simulink model "BESS_Voltage_Controle"  (R2017b)
settings: Solver=ode45  StartTime=0.0  StopTime=5  RelTol=1e-3  EnableMultiTasking=on
values from neighbouring files (symbols this model uses):
  beta = beta (k)    [Parameter_2M_DFIG_BESS.m]
  Cbus = 80e-3    (= 0.08)    [Parameter_2M_DFIG_BESS.m]
  cp_opt_abs = abs(max(Cp))    [Parameter_2M_DFIG_BESS.m]
  D = 0.1    [Parameter_2M_DFIG_BESS.m]
  f = 60    [Parameter_2M_DFIG_BESS.m]
  Fs = 1.8    [Parameter_2M_DFIG_BESS.m]
  fsw = 4e3    (= 4000)    [Parameter_2M_DFIG_BESS.m]
  J = 90    [Parameter_2M_DFIG_BESS.m]
  ki_id = (wni^2)*Lr*sigma    (= 491.599501999)    [Parameter_2M_DFIG_BESS.m]
  ki_idg = (wnig^2)*Lg    (= 68.6450725305)    [Parameter_2M_DFIG_BESS.m]
  ki_iq = ki_id    (= 491.599501999)    [Parameter_2M_DFIG_BESS.m]
  ki_iqg = ki_idg    (= 68.6450725305)    [Parameter_2M_DFIG_BESS.m]
  ki_v = -300000    [Parameter_2M_DFIG_BESS.m]
  kp_id = (2*wni*sigma*Lr)-Rr    (= 0.5771)    [Parameter_2M_DFIG_BESS.m]
  kp_idg = (2*wnig*Lg)-Rg    (= 0.364153420404)    [Parameter_2M_DFIG_BESS.m]
  kp_iq = kp_id    (= 0.5771)    [Parameter_2M_DFIG_BESS.m]
  kp_iqg = kp_idg    (= 0.364153420404)    [Parameter_2M_DFIG_BESS.m]
  kp_v = -1000    [Parameter_2M_DFIG_BESS.m]
  Kpg = 1/(1.5*Vs*sqrt(2/3))    [Parameter_2M_DFIG_BESS.m]
  Kqg = -Kpg    [Parameter_2M_DFIG_BESS.m]
  lambda_opt = abs(lambda(posicion))    [Parameter_2M_DFIG_BESS.m]
  Lg = 483e-6    (= 0.000483)    [Parameter_2M_DFIG_BESS.m]
  Lm = 2.5e-3    (= 0.0025)    [Parameter_2M_DFIG_BESS.m]
  Lr = Lm + Lsr    (= 0.002587)    [Parameter_2M_DFIG_BESS.m]
  Ls = Lm + Lsi    (= 0.002587)    [Parameter_2M_DFIG_BESS.m]
  Lsi = 87e-6    (= 8.7e-05)    [Parameter_2M_DFIG_BESS.m]
  N = 100    [Parameter_2M_DFIG_BESS.m]
  p = 2    [Parameter_2M_DFIG_BESS.m]
  Ps = 2e6    (= 2000000)    [Parameter_2M_DFIG_BESS.m]
  Radio = 44    [Parameter_2M_DFIG_BESS.m]
  Rg = 20e-6    (= 2e-05)    [Parameter_2M_DFIG_BESS.m]
  ro = 1.225    [Parameter_2M_DFIG_BESS.m]
  Rr = 2.9e-3    (= 0.0029)    [Parameter_2M_DFIG_BESS.m]
  Rs = 2.6e-3    (= 0.0026)    [Parameter_2M_DFIG_BESS.m]
  sigma = 1- Lm^2/(Ls*Lr)    (= 0.0661284179513)    [Parameter_2M_DFIG_BESS.m]
  Ts = 1/fsw/f    (= 4.16666666667e-06)    [Parameter_2M_DFIG_BESS.m]
  Vbus_ref = 1200    [Parameter_2M_DFIG_BESS.m]
  Vs = 690    [Parameter_2M_DFIG_BESS.m]
undefined symbols (not defined in the file or in its folder): D1, D11, Delta, DiscIntNeverNeededParam, Ion, Lithium, sigbuilder_block
libraries: powerlib x50, powerlib_meascontrol x21, electricdrivelib x1, simulink x1, sps_avr x1
(part 1 of 2)
settings Model: SimulationMode=accelerator  Creator=admin  LastModifiedBy=admin
settings DataIOCC: LimitDataPoints=on  SaveFormat=Array
settings OptimizationCC: EfficientMapNaN2IntZero=off  LifeSpan=inf
settings DebuggingCC: UnderspecifiedInitializationDetection=Classic  MergeDetectMultiDrivingBlocksExec=none  SolverPrmCheckMsg=warning  StateNameClashWarn=warning  SFUnexpectedBacktrackingDiag=warning  SFNoUnconditionalDefaultTransitionDiag=warning  SFExecutionAtInitializationDiag=none
settings HardwareCC: ProdBitPerPointer=32  ProdBitPerSizeT=32  ProdBitPerPtrDiffT=32  ProdLargestAtomicFloat=None  ProdIntDivRoundTo=Undefined  ProdEndianess=Unspecified  ProdWordSize=32  ProdHWDeviceType=32-bit Generic  TargetBitPerPointer=64  TargetBitPerSizeT=64  TargetBitPerPtrDiffT=64  TargetLongLongMode=on  TargetIntDivRoundTo=Zero  TargetEndianess=LittleEndian  TargetWordSize=64  TargetHWDeviceType=MATLAB Host  ProdEqTarget=off
settings ModelReferenceCC: PropagateSignalLabelsOutOfModel=off
settings CodeAppCC: MaxIdLength=128
settings GRTTargetCC: TargetLangStandard=C89/C90 (ANSI)  CombineOutputUpdateFcns=off  GRTInterface=on
settings ConfigComp: CovMetricSettings=dw  CovHtmlReporting=on  CovSaveCumulativeToWorkspaceVar=on  CovSaveSingleToWorkspaceVar=on  CovExternalEMLEnable=off
settings SimscapeCC: SimscapeNormalizeSystem=off

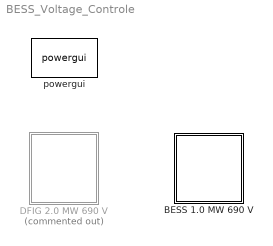
== system BESS_Voltage_Controle ==
  BESS 1.0 MW 690 V : Subsystem
  DFIG 2.0 MW 690 V : Subsystem  Commented=on
  powergui : powerlib/powergui  Priority=1  SimulationMode=Discrete  SampleTime=Ts  frequency=60  Iterations=50  frequencyindice=0  Pbase=100e6  ErrMax=1e-4  UnitsV=kV  UnitsW=MW  buscounter=0  FunctionMessages=off  echomessages=off  EnableUseOfTLC=off  CurrentSourceSwitches=off  DisableSnubberDevices=off  DisableRonSwitches=off  DisableVfSwitches=off  DisplayEquations=off  SolverType=Tustin  Interpol=off  ExternalGateDelay=off  methode=off  Ts=0  x0status=blocks  SPID=off  SwTol=0  HookPort=off  RestoreLinks=warning  ResistiveCurrentMeasurement=off  Frange=[0:2:500]  Ylog=off  Xlog=on  ShowGrid=off  save=off  variable=ZData  structure=0  ZoomFFT=off  StartTime=0.0  cycles=1  DisplayStyle=1  fundamental=60  FreqAxis=off  MaxFrequency=1000  frequencyindicesteady=1  RmsSteady=1  display=off

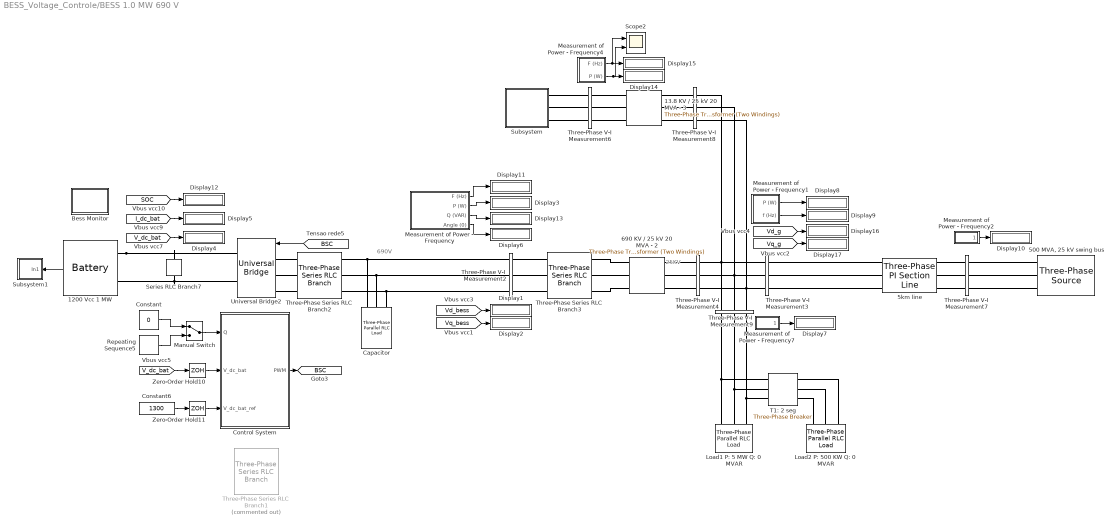
== system BESS_Voltage_Controle/BESS 1.0 MW 690 V ==
  note: 690V
  note: 25KV
  "1200 Vcc 1 MW " : electricdrivelib/Extra Sources/Battery  BatType=Lithium-Ion  ShowTempParam=off  ThermalPreset=no  ShowAgeParam=off  NomV=1200  NomQ=833  SOC=71  Batt_Tr=30  PresetModel=on  MaxQ=833  MinV=900  FullV=1396.7846  Dis_rate=362.1739  R=0.014406  Normal_OP=753.3217  expZone="[1296.463      40.925652]"  current=[833]  Units=Time  Tci=20  NomT=25  T2=0  MaxQ2=2.208  FullV2=3.45  Normal_OP2=2.8  expZone2="[3.22        0.23]"  Rca=0.6  ti=1000  Dp=0  Neq0=0  Tsim=1e6  Ta1=25  Qeol=5.4*0.9  Reol=0.013333*1.2  Char_age=[2.3478, 3]  Dis_age=[2.3478, 10]  N1=1500  N2=10500  N3=1000  N4=1400  Ta2=45  N5=950
  13.8 KV / 25 kV 20 MVA - 3 : powerlib/Elements/Three-Phase Transformer (Two Windings)  Winding1Connection=Delta (D11)  Winding2Connection=Yg  CoreType=Three single-phase transformers  SetSaturation=off  Hysteresis=off  DataFile='hysteresis'  SetInitialFlux=off  Measurements=None  UNITS=SI  NominalPower=[20e6 f]  Winding1=[25000 0.14881 0.011842]  Winding2=[13800 2.624e-05 2.0881e-06]  Rm=89286  Lm=Inf  L0=0.5  Saturation=[0 0;0.47518 112.54;197.99 142.55]  InitialFluxes=[75.026 -75.026 65.648]  MoreParameters=off  BreakLoop=off  DataType=on  TransfoNumber=0
  "500 MVA, 25 kV swing bus" : powerlib/Electrical Sources/Three-Phase Source  InternalConnection=Yg  VoltagePhases=off  Voltage=25e3  PhaseAngle=0  Voltage_phases=[25e3 25e3 25e3]/sqrt(3)  PhaseAngles_phases=[0 -120 +120]  Frequency=f  NonIdealSource=on  SpecifyImpedance=on  Resistance=0  Inductance=47.147e-3  ShortCircuitLevel=500e6  BaseVoltage=25e3  XRratio=100  BusType=swing  Pref=10e3  Qref=0  Prefabc=[10e3, 10e3, 10e3]  Qrefabc=[0, 0, 0]  Qmin=-inf  Qmax=inf
  5km line : powerlib/Elements/Three-Phase PI Section Line  LConnTagsString=a|b|c  RConnTagsString=A|B|C  Frequency=f  Resistances=[0.1153 0.413]  Inductances=[1.05e-3 3.32e-3]  Capacitances=[11.33e-009 5.01e-009]  Length=5
      settings: SourceProductName=Simscape Power Systems
  690 KV / 25 kV 20 MVA - 2 : powerlib/Elements/Three-Phase Transformer (Two Windings)  Winding1Connection=Delta (D11)  Winding2Connection=Yg  CoreType=Three single-phase transformers  SetSaturation=off  Hysteresis=off  DataFile='hysteresis'  SetInitialFlux=off  Measurements=None  UNITS=SI  NominalPower="[20e6  f]"  Winding1=[25000 0.14881 0.011842]  Winding2=[690 2.624e-05 2.0881e-06]  Rm=89286  Lm=Inf  L0=0.5  Saturation=[0 0;0.47518 112.54;197.99 142.55]  InitialFluxes=[75.026 -75.026 65.648]  MoreParameters=off  BreakLoop=off  DataType=on  TransfoNumber=0
  Bess Monitor : Subsystem
  Capacitor : powerlib/Elements/Three-Phase Parallel RLC Load  LConnTagsString=A|B|C  Configuration=Y (grounded)  NominalVoltage=690  Vabc=[1e3 1e3 1e3]  Vabcp=[1e3 1e3 1e3]  NominalFrequency=f  UnbalancedPower=off  ActivePower=0  InductivePower=0  CapacitivePower=15e-3  Pabc=[10e3 9e3 11e3]  QLabc=[100 90 110]  QCabc=[100 90 110]  Pabcp=[10e3 9e3 11e3]  QLabcp=[100 90 110]  QCabcp=[100 90 110]  Measurements=None  LoadType=constant Z
  Constant : Constant  Value=0
  Constant6 : Constant  Value=1300
  Control System : Subsystem
  Display{1..17} (17 alike) : Display
  Load1 P: 5 MW Q: 0 MVAR : powerlib/Elements/Three-Phase Parallel RLC Load  LConnTagsString=A|B|C  Configuration=Y (grounded)  NominalVoltage=25e3  Vabc=[1e3 1e3 1e3]  Vabcp=[1e3 1e3 1e3]  NominalFrequency=f  UnbalancedPower=off  ActivePower=5e6  InductivePower=0  CapacitivePower=0  Pabc=[10e3 9e3 11e3]  QLabc=[100 90 110]  QCabc=[100 90 110]  Pabcp=[10e3 9e3 11e3]  QLabcp=[100 90 110]  QCabcp=[100 90 110]  Measurements=None  LoadType=constant I
  Load2 P: 500 KW Q: 0 MVAR : powerlib/Elements/Three-Phase Parallel RLC Load  LConnTagsString=A|B|C  Configuration=Y (grounded)  NominalVoltage=25e3  Vabc=[1e3 1e3 1e3]  Vabcp=[1e3 1e3 1e3]  NominalFrequency=f  UnbalancedPower=off  ActivePower=500e5  InductivePower=0  CapacitivePower=0  Pabc=[10e3 9e3 11e3]  QLabc=[100 90 110]  QCabc=[100 90 110]  Pabcp=[10e3 9e3 11e3]  QLabcp=[100 90 110]  QCabcp=[100 90 110]  Measurements=None  LoadType=constant I
  Manual Switch : ManualSwitch
  Measurement of Power - Frequency : Subsystem
  Measurement of Power - Frequency1 : Subsystem
  Measurement of Power - Frequency2 : Subsystem
  Measurement of Power - Frequency4 : Subsystem
  Measurement of Power - Frequency7 : Subsystem
  Repeating Sequence5 : simulink/Sources/Repeating Sequence  rep_seq_t=[0 1.499 1.5 2.499 2.5 3.499 3.5 3.999 4 5]  rep_seq_y=[0 0 5e5 5e5 3e5 3e5 -5e5 -5e5 0 0]
  Scope2 : Scope  NumInputPorts=2
  Series RLC Branch7 : powerlib/Elements/Series RLC Branch  LConnTagsString=__new0  RConnTagsString=__new0  BranchType=C  Resistance=1  Inductance=1e-3  SetiL0=off  InitialCurrent=0  Capacitance=15e-3  Setx0=off  InitialVoltage=0  Measurements=Branch voltage
  Subsystem : Subsystem
  Subsystem1 : Subsystem
  "T1: 2 seg " : powerlib/Elements/Three-Phase Breaker  InitialState=open  SwitchA=on  SwitchB=on  SwitchC=on  SwitchTimes=5  External=off  BreakerResistance=0.01  SnubberResistance=1e6  SnubberCapacitance=inf  Measurements=None
  Three-Phase Series RLC Branch1 : powerlib/Elements/Three-Phase Series RLC Branch  Commented=on  LConnTagsString=A|B|C  RConnTagsString=A|B|C  BranchType=RL  Resistance=20e-6  Inductance=483e-6  Capacitance=0  Measurements=None
  Three-Phase Series RLC Branch2 : powerlib/Elements/Three-Phase Series RLC Branch  LConnTagsString=A|B|C  RConnTagsString=A|B|C  BranchType=RL  Resistance=20e-3  Inductance=483e-6  Capacitance=0  Measurements=None
  Three-Phase Series RLC Branch3 : powerlib/Elements/Three-Phase Series RLC Branch  LConnTagsString=A|B|C  RConnTagsString=A|B|C  BranchType=RL  Resistance=20e-3  Inductance=0  Capacitance=0  Measurements=None
  Three-Phase V-I Measurement2 : powerlib/Measurements/Three-Phase V-I Measurement  VoltageMeasurement=phase-to-ground  SetLabelV=on  LabelV=V_ac_bess  Vpu=off  VpuLL=off  CurrentMeasurement=yes  SetLabelI=on  LabelI=I_ac_bess  Ipu=off  Pbase=100e6  Vbase=500e3  OutputType=Complex  PhasorSimulation=off  PSBequivalent=0
  Three-Phase V-I Measurement3 : powerlib/Measurements/Three-Phase V-I Measurement  VoltageMeasurement=phase-to-ground  SetLabelV=on  LabelV=V_ac_line_1  Vpu=off  VpuLL=off  CurrentMeasurement=yes  SetLabelI=on  LabelI=I_ac_line_1  Ipu=off  Pbase=100e6  Vbase=500e3  OutputType=Complex  PhasorSimulation=off  PSBequivalent=0
  Three-Phase V-I Measurement4 : powerlib/Measurements/Three-Phase V-I Measurement  VoltageMeasurement=phase-to-ground  SetLabelV=on  LabelV=V_ac_bat_H  Vpu=off  VpuLL=off  CurrentMeasurement=yes  SetLabelI=on  LabelI=I_ac_bat_H  Ipu=off  Pbase=100e6  Vbase=500e3  OutputType=Complex  PhasorSimulation=off  PSBequivalent=0
  Three-Phase V-I Measurement6 : powerlib/Measurements/Three-Phase V-I Measurement  VoltageMeasurement=phase-to-ground  SetLabelV=on  LabelV=V_ac_syn_low  Vpu=off  VpuLL=off  CurrentMeasurement=yes  SetLabelI=on  LabelI=I_ac_syn_low  Ipu=off  Pbase=100e6  Vbase=500e3  OutputType=Complex  PhasorSimulation=off  PSBequivalent=0
  Three-Phase V-I Measurement7 : powerlib/Measurements/Three-Phase V-I Measurement  VoltageMeasurement=phase-to-ground  SetLabelV=on  LabelV=V_ac_line_2  Vpu=off  VpuLL=off  CurrentMeasurement=yes  SetLabelI=on  LabelI=I_ac_line_2  Ipu=off  Pbase=100e6  Vbase=500e3  OutputType=Complex  PhasorSimulation=off  PSBequivalent=0
  Three-Phase V-I Measurement8 : powerlib/Measurements/Three-Phase V-I Measurement  VoltageMeasurement=phase-to-ground  SetLabelV=on  LabelV=V_ac_syn_H  Vpu=off  VpuLL=off  CurrentMeasurement=yes  SetLabelI=on  LabelI=I_ac_syn_H  Ipu=off  Pbase=100e6  Vbase=500e3  OutputType=Complex  PhasorSimulation=off  PSBequivalent=0
  Three-Phase V-I Measurement9 : powerlib/Measurements/Three-Phase V-I Measurement  VoltageMeasurement=phase-to-ground  SetLabelV=on  LabelV=V_ac_load  Vpu=off  VpuLL=off  CurrentMeasurement=yes  SetLabelI=on  LabelI=I_ac_load  Ipu=off  Pbase=100e6  Vbase=500e3  OutputType=Complex  PhasorSimulation=off  PSBequivalent=0
  Universal Bridge2 : powerlib/Power Electronics/Universal Bridge  Arms=3  SnubberResistance=1e5  SnubberCapacitance=inf  Device=Ideal Switches  Ron=1e-3  Lon=0  ForwardVoltages="[  0  0  ]"  ForwardVoltage=0  GTOparameters=[ 10e-6 , 20e-6 ]  IGBTparameters=[ 1e-6 , 2e-6 ]  Measurements=None  Measurements_2=None  converterType=Rectifier
  Zero-Order Hold10 : ZeroOrderHold  SampleTime=1/fsw
  Zero-Order Hold11 : ZeroOrderHold  SampleTime=1/fsw
  tag scope: BSC=global
  wires:
  Zero-Order Hold10/1 -> Control System/2(V_dc_bat)
  [V_dc_bat] -> Zero-Order Hold10/1
  [I_dc_bat] -> Display5/1
  Control System/1(PWM) -> [BSC]
  Zero-Order Hold11/1 -> Control System/3(V_dc_bat_ref)
  [V_dc_bat] -> Display4/1
  "1200 Vcc 1 MW "/1 -> Subsystem1/1(In1)
  Constant6/1 -> Zero-Order Hold11/1
  [BSC] -> Universal Bridge2/1
  Measurement of Power - Frequency/2(P (W)) -> Display3/1
  Measurement of Power - Frequency/1(F (Hz)) -> Display11/1
  Measurement of Power - Frequency/3(Q (VAR)) -> Display13/1
  [SOC] -> Display12/1
  Manual Switch/1 -> Control System/1(Q)
  Constant/1 -> Manual Switch/1
  Repeating Sequence5/1 -> Manual Switch/2
  [Vd_bess] -> Display1/1
  [Vq_bess] -> Display2/1
  Measurement of Power - Frequency/4(Angle (0)) -> Display6/1
  Measurement of Power - Frequency7/1(P (W)) -> Display7/1
  Measurement of Power - Frequency2/1(P (W)) -> Display10/1
  Measurement of Power - Frequency1/1(P (W)) -> Display8/1
  Measurement of Power - Frequency4/2(P (W)) -> Display14/1, Scope2/2
  Measurement of Power - Frequency4/1(F (Hz)) -> Scope2/1, Display15/1
  [Vd_g] -> Display16/1
  [Vq_g] -> Display17/1
  Measurement of Power - Frequency1/2(f (Hz)) -> Display9/1
  connections:
  Series RLC Branch7/RConn1 -- "1200 Vcc 1 MW "/LConn2 -- Universal Bridge2/RConn2
  "1200 Vcc 1 MW "/LConn1 -- Series RLC Branch7/LConn1 -- Universal Bridge2/RConn1
  Capacitor/LConn1 -- Three-Phase V-I Measurement2/LConn1 -- Three-Phase Series RLC Branch2/RConn1
  Capacitor/LConn2 -- Three-Phase Series RLC Branch2/RConn2 -- Three-Phase V-I Measurement2/LConn2
  Capacitor/LConn3 -- Three-Phase V-I Measurement2/LConn3 -- Three-Phase Series RLC Branch2/RConn3
  Load1 P: 5 MW Q: 0 MVAR/LConn1 -- Three-Phase V-I Measurement9/RConn3 -- "T1: 2 seg "/LConn1
  Load1 P: 5 MW Q: 0 MVAR/LConn2 -- Three-Phase V-I Measurement9/RConn2 -- "T1: 2 seg "/LConn2
  Load1 P: 5 MW Q: 0 MVAR/LConn3 -- Three-Phase V-I Measurement9/RConn1 -- "T1: 2 seg "/LConn3
  690 KV / 25 kV 20 MVA - 2/LConn2 -- Three-Phase V-I Measurement4/LConn2
  690 KV / 25 kV 20 MVA - 2/LConn3 -- Three-Phase V-I Measurement4/LConn3
  690 KV / 25 kV 20 MVA - 2/LConn1 -- Three-Phase V-I Measurement4/LConn1
  5km line/RConn1 -- Three-Phase V-I Measurement7/LConn1
  5km line/LConn1 -- Three-Phase V-I Measurement3/RConn1
  5km line/LConn2 -- Three-Phase V-I Measurement3/RConn2
  5km line/RConn2 -- Three-Phase V-I Measurement7/LConn2
  5km line/RConn3 -- Three-Phase V-I Measurement7/LConn3
  5km line/LConn3 -- Three-Phase V-I Measurement3/RConn3
  "500 MVA, 25 kV swing bus"/RConn1 -- Three-Phase V-I Measurement7/RConn1
  "500 MVA, 25 kV swing bus"/RConn2 -- Three-Phase V-I Measurement7/RConn2
  "500 MVA, 25 kV swing bus"/RConn3 -- Three-Phase V-I Measurement7/RConn3
  Three-Phase V-I Measurement4/RConn1 -- Three-Phase V-I Measurement8/RConn1 -- Three-Phase V-I Measurement9/LConn3 -- Three-Phase V-I Measurement3/LConn1
  Three-Phase V-I Measurement4/RConn2 -- Three-Phase V-I Measurement8/RConn2 -- Three-Phase V-I Measurement9/LConn2 -- Three-Phase V-I Measurement3/LConn2
  Three-Phase V-I Measurement4/RConn3 -- Three-Phase V-I Measurement8/RConn3 -- Three-Phase V-I Measurement3/LConn3 -- Three-Phase V-I Measurement9/LConn1
  Load2 P: 500 KW Q: 0 MVAR/LConn1 -- "T1: 2 seg "/RConn3
  Load2 P: 500 KW Q: 0 MVAR/LConn2 -- "T1: 2 seg "/RConn2
  Load2 P: 500 KW Q: 0 MVAR/LConn3 -- "T1: 2 seg "/RConn1
  Subsystem/LConn2 -- Three-Phase V-I Measurement6/LConn2
  Three-Phase V-I Measurement8/LConn3 -- 13.8 KV / 25 kV 20 MVA - 3/LConn3
  Subsystem/LConn3 -- Three-Phase V-I Measurement6/LConn3
  Subsystem/LConn1 -- Three-Phase V-I Measurement6/LConn1
  Three-Phase V-I Measurement8/LConn2 -- 13.8 KV / 25 kV 20 MVA - 3/LConn2
  Three-Phase V-I Measurement6/RConn3 -- 13.8 KV / 25 kV 20 MVA - 3/RConn3
  Three-Phase V-I Measurement6/RConn2 -- 13.8 KV / 25 kV 20 MVA - 3/RConn2
  Three-Phase V-I Measurement6/RConn1 -- 13.8 KV / 25 kV 20 MVA - 3/RConn1
  Three-Phase V-I Measurement8/LConn1 -- 13.8 KV / 25 kV 20 MVA - 3/LConn1
  Three-Phase Series RLC Branch2/LConn1 -- Universal Bridge2/LConn1
  Three-Phase Series RLC Branch2/LConn2 -- Universal Bridge2/LConn2
  Three-Phase Series RLC Branch2/LConn3 -- Universal Bridge2/LConn3
  Three-Phase Series RLC Branch3/LConn1 -- Three-Phase V-I Measurement2/RConn1
  Three-Phase Series RLC Branch3/LConn2 -- Three-Phase V-I Measurement2/RConn2
  Three-Phase Series RLC Branch3/LConn3 -- Three-Phase V-I Measurement2/RConn3
  Three-Phase Series RLC Branch3/RConn1 -- 690 KV / 25 kV 20 MVA - 2/RConn1
  Three-Phase Series RLC Branch3/RConn2 -- 690 KV / 25 kV 20 MVA - 2/RConn2
  Three-Phase Series RLC Branch3/RConn3 -- 690 KV / 25 kV 20 MVA - 2/RConn3

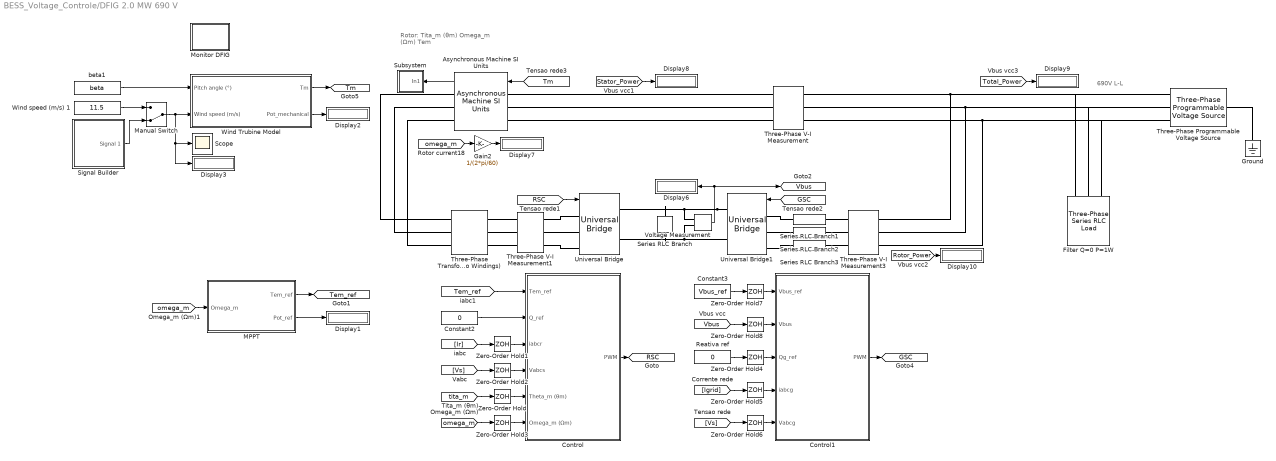
== system BESS_Voltage_Controle/DFIG 2.0 MW 690 V ==
  note: 690V L-L
  note: Rotor:
      | Tita_m (θm)
      | Omega_m (Ωm)
      | Tem
  Asynchronous Machine SI Units : powerlib/Machines/Asynchronous Machine SI Units  RotorType=Wound  PresetModel=No  MechanicalLoad=Torque Tm  ShowDetailedParameters=on  ReferenceFrame=Rotor  Units=SI  MeasurementBus=off  NominalParameters=[ Ps Vs f ]  Stator=[ Rs , Lsi]  Rotor=[ Rr , Lsi]  Cage1=[ 0.022 0.226/377]  Cage2=[ 0.022 0.226/377]  Lm=Lm  Mechanical=[ J D 2 ]  PolePairs=2  InitialConditions=[1 0 0 0 0 0 0 0]  SimulateSaturation=off  Saturation=[14.03593122, 27.81365428, 53.79336849, 72.68890987, 97.98006896, 148.6815601, 215.7428561, 302.9841135, 420.4778367 ; 230, 322, 414, 460, 506, 552, 598, 644, 690]  LoadFlowParameters=1492000  TsPowergui=0  TsBlock=-1  IterativeModel=Trapezoidal non iterative  IterativeDiscreteModel=Trapezoidal non iterative  Pmec=0
  Constant2 : Constant  Value=0
  Constant3 : Constant  Value=Vbus_ref
  Control : Subsystem
  Control1 : Subsystem
  Display{1..3,6..10} (8 alike) : Display
  Filter Q=0 P=1W : powerlib/Elements/Three-Phase Series RLC Load  LConnTagsString=A|B|C  Configuration=Y (grounded)  NominalVoltage=Vs  Vabc=[1e3 1e3 1e3]  Vabcp=[1e3 1e3 1e3]  NominalFrequency=f  UnbalancedPower=off  ActivePower=1  InductivePower=0  CapacitivePower=0  Pabc=[10e3 9e3 11e3]  QLabc=[100 90 110]  QCabc=[100 90 110]  Pabcp=[10e3 9e3 11e3]  QLabcp=[100 90 110]  QCabcp=[100 90 110]  Measurements=None  LoadType=constant Z
  Gain2 : Gain  Gain=1/(2*pi/60)
  Ground : powerlib/Elements/Ground  LConnTagsString=a
  MPPT : Subsystem
  Manual Switch : ManualSwitch  CurrentSetting=0
  Monitor DFIG : Subsystem
  Reativa ref : Constant  Value=0
  Scope : Scope
  Series RLC Branch : powerlib/Elements/Series RLC Branch  LConnTagsString=__new0  RConnTagsString=__new0  BranchType=C  Resistance=1  Inductance=1e-3  SetiL0=off  InitialCurrent=0  Capacitance=Cbus  Setx0=off  InitialVoltage=0  Measurements=Branch voltage
  Series RLC Branch1 : powerlib/Elements/Series RLC Branch  LConnTagsString=__new0  RConnTagsString=__new0  BranchType=RL  Resistance=Rg  Inductance=Lg  SetiL0=off  InitialCurrent=0  Capacitance=0  Setx0=off  InitialVoltage=0  Measurements=None
  Series RLC Branch2 : powerlib/Elements/Series RLC Branch  LConnTagsString=__new0  RConnTagsString=__new0  BranchType=RL  Resistance=Rg  Inductance=Lg  SetiL0=off  InitialCurrent=0  Capacitance=0  Setx0=off  InitialVoltage=0  Measurements=None
  Series RLC Branch3 : powerlib/Elements/Series RLC Branch  LConnTagsString=__new0  RConnTagsString=__new0  BranchType=RL  Resistance=Rg  Inductance=Lg  SetiL0=off  InitialCurrent=0  Capacitance=0  Setx0=off  InitialVoltage=0  Measurements=None
  Signal Builder : Subsystem  Tag=STV Subsys  LoadFcn=sigbuilder_block('load');  StartFcn=sigbuilder_block('start');  StopFcn=sigbuilder_block('stop');  ClipboardFcn=sigbuilder_block('clipboard');  mask(Sigbuilder block){tuvar=[0:10]}
      mask help: Simulink:masks:SigbuilderBlock_MD
      mask init:
      | if ~strcmp(get_param(bdroot(gcbh),'SimulationStatus'),'stopped') tuvar = sigbuilder_block('maskInit'); end
      settings: CopyFcn=sigbuilder_block('copy');  DeleteFcn=sigbuilder_block('delete');  ModelCloseFcn=sigbuilder_block('modelClose');  PreSaveFcn=sigbuilder_block('preSave');  PauseFcn=sigbuilder_block('pause');  ContinueFcn=sigbuilder_block('continue');  NameChangeFcn=sigbuilder_block('namechange');  OpenFcn=sigbuilder_block('open',[6 22.5 1012.5 455.25 ]);  CloseFcn=sigbuilder_block('close');
      mask Display: plot(0, 0, 100, 100,[2, 2, 32, 32, 2], [68, 8, 8, 68, 68],[32, 2], [38, 38], [32, 19, 2],[53, 60, 44], [32, 17, 17, 2],[16, 16, 31, 31]);txt = getActiveGroup(gcbh);text(2, 100, txt,'verticalAlignment', 'top');
  Subsystem : Subsystem
  Three-Phase Programmable Voltage Source : powerlib/Electrical Sources/Three-Phase Programmable Voltage Source  PositiveSequence="[Vs  0 f]"  VariationEntity=Frequency  VariationType=Table of time-amplitude pairs  VariationTypeAlt=Step  VariationStep=-0.8  VariationRate=10  VariationMagnitude=0.3  VariationFrequency=2  VariationTiming=[0.2 3]  VariationPhaseA=off  Amplitudes=[1 0.8 1.2 1.0]  TimeValues=[0 0.1 0.15 0.2]  HarmonicGeneration=off  HarmonicA=[3 0.2 -25 0]  HarmonicB=[2 0.15 35 2]  Timing="[0.05  3]"  BusType=swing  Pref=0  Qref=0  Qmin=-inf  Qmax=inf
  Three-Phase Transformer (Two Windings) : powerlib/Elements/Three-Phase Transformer (Two Windings)  Winding1Connection=Y  Winding2Connection=Y  CoreType=Three single-phase transformers  SetSaturation=off  Hysteresis=off  DataFile='hysteresis'  SetInitialFlux=off  Measurements=None  UNITS=SI  NominalPower=[ Ps , f]  Winding1=[Vs 0 0]  Winding2=[Vs/u 0 0]  Rm=1.0805e+06  Lm=2866  L0=0.5  Saturation=[0 0;0.66653 1910.3;277.72 2419.7]  InitialFluxes=[1273.5 -1273.5 1114.3]  MoreParameters=off  BreakLoop=off  DataType=on  TransfoNumber=1
  Three-Phase V-I Measurement : powerlib/Measurements/Three-Phase V-I Measurement  VoltageMeasurement=phase-to-ground  SetLabelV=on  LabelV=Vs  Vpu=off  VpuLL=off  CurrentMeasurement=yes  SetLabelI=on  LabelI=Is  Ipu=off  Pbase=100e6  Vbase=500e3  OutputType=Complex  PhasorSimulation=off  PSBequivalent=0
  Three-Phase V-I Measurement1 : powerlib/Measurements/Three-Phase V-I Measurement  VoltageMeasurement=phase-to-phase  SetLabelV=on  LabelV=Vr  Vpu=off  VpuLL=off  CurrentMeasurement=yes  SetLabelI=on  LabelI=Ir  Ipu=off  Pbase=100e6  Vbase=500e3  OutputType=Complex  PhasorSimulation=off  PSBequivalent=0
  Three-Phase V-I Measurement3 : powerlib/Measurements/Three-Phase V-I Measurement  VoltageMeasurement=phase-to-ground  SetLabelV=on  LabelV=Vgrid  Vpu=off  VpuLL=off  CurrentMeasurement=yes  SetLabelI=on  LabelI=Igrid  Ipu=off  Pbase=100e6  Vbase=500e3  OutputType=Complex  PhasorSimulation=off  PSBequivalent=0
  Universal Bridge : powerlib/Power Electronics/Universal Bridge  Arms=3  SnubberResistance=1e5  SnubberCapacitance=inf  Device=Ideal Switches  Ron=1e-3  Lon=0  ForwardVoltages="[  0  0  ]"  ForwardVoltage=0  GTOparameters=[ 10e-6 , 20e-6 ]  IGBTparameters=[ 1e-6 , 2e-6 ]  Measurements=None  Measurements_2=None  converterType=Rectifier
  Universal Bridge1 : powerlib/Power Electronics/Universal Bridge  Arms=3  SnubberResistance=1e5  SnubberCapacitance=inf  Device=Ideal Switches  Ron=1e-3  Lon=0  ForwardVoltages="[  0  0  ]"  ForwardVoltage=0  GTOparameters=[ 10e-6 , 20e-6 ]  IGBTparameters=[ 1e-6 , 2e-6 ]  Measurements=None  Measurements_2=None  converterType=Rectifier
  Voltage Measurement : powerlib/Measurements/Voltage Measurement  PhasorSimulation=off  OutputType=Complex  PSBequivalent=0
  Wind Trubine Model : Subsystem
  Wind speed (m/s) 1 : Constant  Value=11.5
  Zero-Order Hold{,1..8} (9 alike) : ZeroOrderHold  SampleTime=1/fsw
  beta1 : Constant  Value=beta
  tag scope: GSC=global, RSC=global, Tem_ref=global, Tm=global, Vbus=global
  wires:
  [Igrid] -> Zero-Order Hold5/1
  beta1/1 -> Wind Trubine Model/1(Pitch angle (°))
  Constant3/1 -> Zero-Order Hold7/1
  MPPT/1(Tem_ref) -> [Tem_ref]
  Wind Trubine Model/1(Tm) -> [Tm]
  [Stator_Power] -> Display8/1
  [Tm] -> Asynchronous Machine SI Units/1
  MPPT/2("Pot_ref ") -> Display1/1
  Reativa ref/1 -> Zero-Order Hold4/1
  [GSC] -> Universal Bridge1/1
  Wind Trubine Model/2(Pot_mechanical) -> Display2/1
  [omega_m] -> MPPT/1(Omega_m)
  Control/1(PWM) -> [RSC]
  [tita_m] -> Zero-Order Hold/1
  [Tem_ref] -> Control/1(Tem_ref)
  [Rotor_Power] -> Display10/1
  [omega_m] -> Gain2/1
  [Vs] -> Zero-Order Hold2/1
  Asynchronous Machine SI Units/1 -> Subsystem/1(In1)
  Zero-Order Hold/1 -> Control/5(Theta_m (θm))
  Zero-Order Hold2/1 -> Control/4(Vabcs)
  [omega_m] -> Zero-Order Hold3/1
  Gain2/1 -> Display7/1
  Zero-Order Hold1/1 -> Control/3(iabcr)
  Constant2/1 -> Control/2(Q_ref)
  [Vbus] -> Zero-Order Hold8/1
  Zero-Order Hold7/1 -> Control1/1(Vbus_ref)
  [RSC] -> Universal Bridge/1
  Zero-Order Hold3/1 -> Control/6("Omega_m (Ωm) ")
  [Ir] -> Zero-Order Hold1/1
  [Vs] -> Zero-Order Hold6/1
  [Total_Power] -> Display9/1
  Zero-Order Hold6/1 -> Control1/5("Vabcg ")
  Zero-Order Hold5/1 -> Control1/4(iabcg)
  Voltage Measurement/1 -> Display6/1, [Vbus]
  Zero-Order Hold4/1 -> Control1/3(Qg_ref)
  Control1/1(PWM) -> [GSC]
  Zero-Order Hold8/1 -> Control1/2(Vbus)
  Manual Switch/1 -> Display3/1, Scope/1, Wind Trubine Model/2(Wind speed (m/s))
  Wind speed (m/s) 1/1 -> Manual Switch/1
  Signal Builder/1(Signal 1) -> Manual Switch/2
  connections:
  Three-Phase V-I Measurement/RConn2 -- Three-Phase Programmable Voltage Source/RConn2 -- Filter Q=0 P=1W/LConn2 -- Three-Phase V-I Measurement3/RConn2
  Three-Phase V-I Measurement/RConn1 -- Three-Phase Programmable Voltage Source/RConn1 -- Filter Q=0 P=1W/LConn1 -- Three-Phase V-I Measurement3/RConn1
  Voltage Measurement/LConn2 -- Universal Bridge1/RConn2 -- Universal Bridge/RConn2 -- Series RLC Branch/RConn1
  Universal Bridge1/RConn1 -- Voltage Measurement/LConn1 -- Universal Bridge/RConn1 -- Series RLC Branch/LConn1
  Three-Phase V-I Measurement/RConn3 -- Three-Phase Programmable Voltage Source/RConn3 -- Filter Q=0 P=1W/LConn3 -- Three-Phase V-I Measurement3/RConn3
  Three-Phase Transformer (Two Windings)/LConn2 -- Asynchronous Machine SI Units/RConn2
  Three-Phase Transformer (Two Windings)/LConn3 -- Asynchronous Machine SI Units/RConn3
  Three-Phase V-I Measurement3/LConn2 -- Series RLC Branch2/RConn1
  Three-Phase V-I Measurement1/LConn1 -- Universal Bridge/LConn1
  Three-Phase V-I Measurement/LConn1 -- Asynchronous Machine SI Units/LConn1
  Three-Phase V-I Measurement3/LConn3 -- Series RLC Branch3/RConn1
  Three-Phase Transformer (Two Windings)/LConn1 -- Asynchronous Machine SI Units/RConn1
  Three-Phase V-I Measurement/LConn3 -- Asynchronous Machine SI Units/LConn3
  Three-Phase V-I Measurement3/LConn1 -- Series RLC Branch1/RConn1
  Three-Phase Transformer (Two Windings)/RConn3 -- Three-Phase V-I Measurement1/RConn3
  Three-Phase V-I Measurement1/LConn3 -- Universal Bridge/LConn3
  Universal Bridge1/LConn1 -- Series RLC Branch1/LConn1
  Three-Phase V-I Measurement1/LConn2 -- Universal Bridge/LConn2
  Three-Phase Transformer (Two Windings)/RConn2 -- Three-Phase V-I Measurement1/RConn2
  Universal Bridge1/LConn3 -- Series RLC Branch3/LConn1
  Three-Phase V-I Measurement/LConn2 -- Asynchronous Machine SI Units/LConn2
  Universal Bridge1/LConn2 -- Series RLC Branch2/LConn1
  Three-Phase Transformer (Two Windings)/RConn1 -- Three-Phase V-I Measurement1/RConn1
  Ground/LConn1 -- Three-Phase Programmable Voltage Source/LConn1

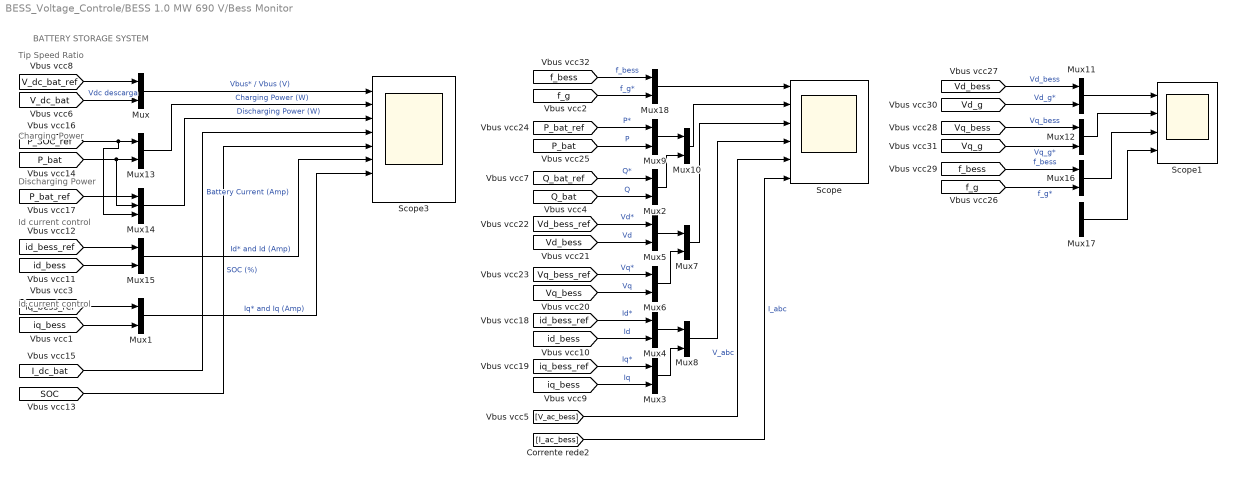
== system BESS_Voltage_Controle/BESS 1.0 MW 690 V/Bess Monitor ==
  note: BATTERY STORAGE SYSTEM
  note: Tip Speed Ratio
  note: Charging Power
  note: Discharging Power
  note: Id current control
  note: Id current control
  Mux{,1..13,15..18} (18 alike) : Mux  Inputs=2
  Mux14 : Mux  Inputs=3
  Scope : Scope  NumInputPorts=6
  Scope1 : Scope  NumInputPorts=4
  Scope3 : Scope  NumInputPorts=8
  wires:
  [P_bat_ref] -> Mux14/1
  Mux13/1 -> Scope3/2  "Charging Power (W)"
  [P_SOC_ref] -> Mux14/3, Mux13/1
  [P_bat] -> Mux14/2, Mux13/2
  [id_bess_ref] -> Mux15/1
  [V_dc_bat_ref] -> Mux/1
  Mux/1 -> Scope3/1  "Vbus* / Vbus (V)"
  [id_bess] -> Mux15/2
  Mux14/1 -> Scope3/3  "Discharging Power (W)"
  [SOC] -> Scope3/5  "SOC (%)"
  [I_dc_bat] -> Scope3/4  "Battery Current (Amp)"
  Mux15/1 -> Scope3/6  "Id* and Id (Amp)"
  [V_dc_bat] -> Mux/2  "Vdc descarga"
  [iq_bess] -> Mux1/2
  [iq_bess_ref] -> Mux1/1
  Mux1/1 -> Scope3/7  "Iq* and Iq (Amp)"
  [Q_bat_ref] -> Mux2/1  "Q*"
  [Q_bat] -> Mux2/2  "Q"
  [iq_bess_ref] -> Mux3/1  "Iq*"
  [id_bess] -> Mux4/2  "Id"
  [iq_bess] -> Mux3/2  "Iq"
  [id_bess_ref] -> Mux4/1  "Id*"
  [Vq_bess_ref] -> Mux6/1  "Vq*"
  [Vq_bess] -> Mux6/2  "Vq"
  Mux4/1 -> Mux8/1
  Mux6/1 -> Mux7/2
  Mux5/1 -> Mux7/1
  Mux7/1 -> Scope/3
  Mux3/1 -> Mux8/2
  Mux8/1 -> Scope/4
  [V_ac_bess] -> Scope/5  "V_abc"
  [I_ac_bess] -> Scope/6  "I_abc"
  [P_bat_ref] -> Mux9/1  "P*"
  [P_bat] -> Mux9/2  "P"
  Mux9/1 -> Mux10/1
  Mux2/1 -> Mux10/2
  Mux10/1 -> Scope/2
  [Vd_bess] -> Mux5/2  "Vd"
  [Vd_bess_ref] -> Mux5/1  "Vd*"
  [Vq_g] -> Mux12/2  "Vq_g*"
  [Vq_bess] -> Mux12/1  "Vq_bess"
  [Vd_bess] -> Mux11/1  "Vd_bess"
  Mux17/1 -> Scope1/4
  [Vd_g] -> Mux11/2  "Vd_g*"
  Mux11/1 -> Scope1/1
  Mux16/1 -> Scope1/3
  [f_bess] -> Mux16/1  "f_bess"
  [f_g] -> Mux16/2  "f_g*"
  Mux12/1 -> Scope1/2
  [f_bess] -> Mux18/1  "f_bess"
  [f_g] -> Mux18/2  "f_g*"
  Mux18/1 -> Scope/1

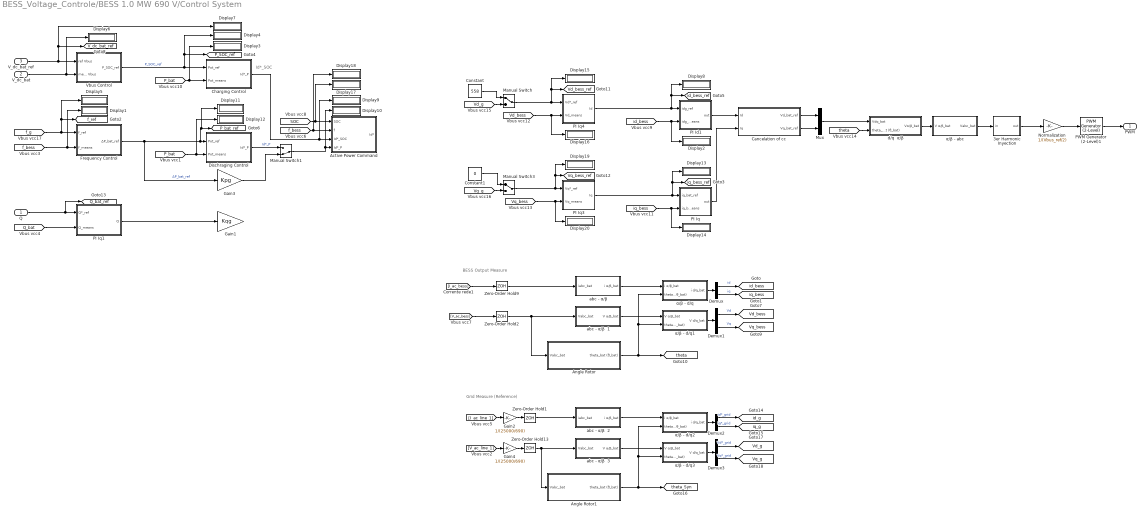
== system BESS_Voltage_Controle/BESS 1.0 MW 690 V/Control System ==
  note: BESS Output Measure
  note: Id*_SOC
  note: Grid Measure (Reference)
  Q : Inport
  V_dc_bat : Inport  Port=2
  V_dc_bat_ref : Inport  Port=3
  " Angle Rotor" : Subsystem
  " Angle Rotor1" : Subsystem
  3er Harmonic Inyection : Subsystem
  Active Power Command : Subsystem
  Cancelation of cc : Subsystem
  Charging Control : Subsystem
  Constant : Constant  Value=558
  Constant1 : Constant  Value=0
  Demux{,1..3} (4 alike) : Demux  Outputs=2
  Dischraging Control : Subsystem
  Display{1..20} (20 alike) : Display
  Frequency Control : Subsystem
  Gain1 : Gain  Gain=Kqg
  Gain2 : Gain  Gain=1/(25000/690)
  Gain3 : Gain  Gain=Kpg
  Gain4 : Gain  Gain=1/(25000/690)
  Manual Switch : ManualSwitch
  Manual Switch1 : ManualSwitch  CurrentSetting=0
  Manual Switch3 : ManualSwitch
  Mux : Mux  Inputs=2
  Normalization : Gain  Gain=1/(Vbus_ref/2)
  PI Id1 : Subsystem
  PI Iq : Subsystem
  PI Iq1 : Subsystem
  PI Iq3 : Subsystem
  PI Iq4 : Subsystem
  PWM Generator (2-Level)1 : powerlib_meascontrol/Pulse & Signal Generators/PWM Generator (2-Level)  ModulatorType=Three-phase bridge (6 pulses)  ModulatorMode=Unsynchronized  Fc=fsw  Pc=0  nF=27  MinMax="[ -1  1 ]"  SamplingTechnique=Natural  ModulatingSignals=off  m=0.8  Freq=60  Phase=0  Ts=0  ShowCarrierOutport=off
      settings: SourceProductName=Simscape Power Systems
  Vbus Control : Subsystem
  Zero-Order Hold{1..2,9,13} (4 alike) : ZeroOrderHold  SampleTime=1/fsw
  "abc - α/β  " : Subsystem
  abc - α/β  1 : Subsystem
  abc - α/β  2 : Subsystem
  abc - α/β  3 : Subsystem
  "d/q  α/β " : Subsystem
  α/β - abc : Subsystem
  α/β - d/q : Subsystem
  α/β - d/q1 : Subsystem
  α/β - d/q2 : Subsystem
  α/β - d/q3 : Subsystem
  PWM : Outport
  tag scope: P_SOC_ref=global, P_bat_ref=global, Q_bat_ref=global, V_dc_bat_ref=global, Vd_bess=global, Vd_bess_ref=global, Vd_g=global, Vq_bess=global, Vq_bess_ref=global, Vq_g=global, f_ref=global, id_bess=global, id_bess_ref=global, id_g=global, iq_bess=global, iq_bess_ref=global, iq_g=global, theta=global, theta_Syn=global
  wires:
  PWM Generator (2-Level)1/1 -> PWM/1
  α/β - d/q/1(i d/q_bat) -> Demux/1
  Zero-Order Hold2/1 -> " Angle Rotor"/1(Vabc_bat), abc - α/β  1/1(Vabc_bat)
  α/β - abc/1(Vabc_bat) -> 3er Harmonic Inyection/1(in)
  Zero-Order Hold9/1 -> "abc - α/β  "/1(iabc_bat)
  "d/q  α/β "/1("Vα/β_bat ") -> α/β - abc/1(V α/β_bat)
  "abc - α/β  "/1(i α/β_bat) -> α/β - d/q/1(i α/β_bat)
  3er Harmonic Inyection/1(out) -> Normalization/1
  PI Id1/1(out) -> Cancelation of cc/1(Id)
  PI Iq/1("out ") -> Cancelation of cc/2(Iq)
  Normalization/1 -> PWM Generator (2-Level)1/1
  V_dc_bat/1 -> Display6/1, Vbus Control/2("means Vbus ")
  [f_g] -> Frequency Control/1(f_ref), [f_ref], Display5/1
  [P_bat] -> Display12/1, Dischraging Control/2("Pot_means ")
  [f_bess] -> Display1/1, Frequency Control/2(f_means)
  [f_bess] -> Active Power Command/2(f), Display18/1
  [SOC] -> Active Power Command/1(SOC), Display17/1
  V_dc_bat_ref/1 -> [V_dc_bat_ref], Display7/1, Vbus Control/1("ref Vbus ")
  Charging Control/1(Id*_P) -> Display9/1, Active Power Command/3(Id*_SOC)
  Vbus Control/1(P_SOC_ref) -> [P_SOC_ref], Display4/1, Charging Control/1("Pot_ref ")  "P_SOC_ref"
  [P_bat] -> Charging Control/2("Pot_means "), Display3/1
  [Q_bat] -> PI Iq1/2(Q_means)
  Demux1/1 -> [Vd_bess]  "Vd"
  abc - α/β  1/1(V α/β_bat) -> α/β - d/q1/1(V α/β_bat)
  α/β - d/q1/1(V d/q_bat) -> Demux1/1
  Demux1/2 -> [Vq_bess]  "Vq"
  Q/1 -> [Q_bat_ref], PI Iq1/1(Q*_ref)
  Mux/1 -> "d/q  α/β "/1(Vdq_bat)
  PI Iq1/1("Q ") -> Gain1/1
  Cancelation of cc/1(" Vd_bat_ref") -> Mux/1
  Cancelation of cc/2(" Vq_bat_ref") -> Mux/2
  " Angle Rotor"/1(theta_bat (θ_bat)) -> α/β - d/q1/2(theta_bat (θ_bat)), α/β - d/q/2(theta_bat (θ_bat)), [theta]
  Demux/1 -> [id_bess]  "id"
  Demux/2 -> [iq_bess]  "iq"
  [theta] -> "d/q  α/β "/2(theta_bat (θ_bat))
  [id_bess] -> PI Id1/2(idg_means), Display2/1
  [iq_bess] -> Display14/1, PI Iq/2(iq_bat_means)
  Manual Switch/1 -> Display15/1, [Vd_bess_ref], PI Iq4/1(Vd*_ref)
  Constant/1 -> Manual Switch/1
  [Vd_bess] -> Display16/1, PI Iq4/2(Vd_means)
  [Vq_bess] -> Display20/1, PI Iq3/2(Vq_means)
  Manual Switch3/1 -> Display19/1, [Vq_bess_ref], PI Iq3/1(Vq*_ref)
  Constant1/1 -> Manual Switch3/1
  Frequency Control/1("ΔP_bat_ref ") -> Dischraging Control/1("Pot_ref "), Display11/1, [P_bat_ref], Gain3/1  "ΔP_bat_ref"
  Dischraging Control/1(Id*_P) -> Manual Switch1/1  "Id*_P"
  Gain3/1 -> Manual Switch1/2
  Manual Switch1/1 -> Active Power Command/4(Id*_P), Display10/1
  PI Iq3/1("Iq ") -> Display13/1, [iq_bess_ref], PI Iq/1(iq_bat_ref)
  PI Iq4/1("Id ") -> Display8/1, [id_bess_ref], PI Id1/1(idg_ref)
  Demux3/2 -> [Vq_g]  "Vq*_grid"
  Demux3/1 -> [Vd_g]  "Vd*_grid"
  abc - α/β  3/1(V α/β_bat) -> α/β - d/q3/1(V α/β_bat)
  abc - α/β  2/1(i α/β_bat) -> α/β - d/q2/1(i α/β_bat)
  " Angle Rotor1"/1(theta_bat (θ_bat)) -> α/β - d/q3/2(theta_bat (θ_bat)), α/β - d/q2/2(theta_bat (θ_bat)), [theta_Syn]
  Demux2/1 -> [id_g]  "id*_grid"
  Demux2/2 -> [iq_g]  "iq*_grid"
  α/β - d/q2/1(i d/q_bat) -> Demux2/1
  α/β - d/q3/1(V d/q_bat) -> Demux3/1
  [I_ac_line_1] -> Gain2/1
  Gain2/1 -> Zero-Order Hold1/1
  [V_ac_line_1] -> Gain4/1
  Gain4/1 -> Zero-Order Hold13/1
  Zero-Order Hold1/1 -> abc - α/β  2/1(iabc_bat)
  Zero-Order Hold13/1 -> " Angle Rotor1"/1(Vabc_bat), abc - α/β  3/1(Vabc_bat)
  [Vd_g] -> Manual Switch/2
  [Vq_g] -> Manual Switch3/2
  [I_ac_bess] -> Zero-Order Hold9/1
  [V_ac_bess] -> Zero-Order Hold2/1

== system BESS_Voltage_Controle/BESS 1.0 MW 690 V/Measurement of Power - Frequency ==
  PLL (3ph)1 : powerlib_meascontrol/PLL/PLL (3ph)  Fmin=45  Par_Init=[0, f]  ParK=[180, 3200, 1]  TcD=1e-4  MaxRateChangeFreq=12  FilterCutOffFreq=25  Ts=0  AGC=on
  "Power (3ph, Instantaneous)1" : powerlib_meascontrol/Measurements/Power (3ph, Instantaneous)
      settings: SourceProductName=Simscape Power Systems
  F (Hz) : Outport
  P (W) : Outport  Port=2
  Q (VAR) : Outport  Port=3
  Angle (0) : Outport  Port=4
  tag scope: P_bat=global, Q_bat=global, f_bess=global, wt_mean=global
  wires:
  [V_ac_bess] -> "Power (3ph, Instantaneous)1"/1, PLL (3ph)1/1
  "Power (3ph, Instantaneous)1"/1 -> P (W)/1, [P_bat]  "Pot"
  PLL (3ph)1/1 -> F (Hz)/1, [f_bess]
  [I_ac_bess] -> "Power (3ph, Instantaneous)1"/2
  "Power (3ph, Instantaneous)1"/2 -> Q (VAR)/1, [Q_bat]
  PLL (3ph)1/2 -> Angle (0)/1, [wt_mean]

== system BESS_Voltage_Controle/BESS 1.0 MW 690 V/Measurement of Power - Frequency1 ==
  PLL (3ph)1 : powerlib_meascontrol/PLL/PLL (3ph)  Fmin=45  Par_Init=[0, f]  ParK=[180, 3200, 1]  TcD=1e-4  MaxRateChangeFreq=12  FilterCutOffFreq=25  Ts=0  AGC=on
  "Power (3ph, Instantaneous)1" : powerlib_meascontrol/Measurements/Power (3ph, Instantaneous)
      settings: SourceProductName=Simscape Power Systems
  P (W) : Outport
  f (Hz) : Outport  Port=2
  tag scope: f_g=global
  wires:
  [V_ac_line_1] -> PLL (3ph)1/1, "Power (3ph, Instantaneous)1"/1
  "Power (3ph, Instantaneous)1"/1 -> P (W)/1  "Pot"
  [I_ac_line_1] -> "Power (3ph, Instantaneous)1"/2
  PLL (3ph)1/1 -> [f_g], f (Hz)/1

== system BESS_Voltage_Controle/BESS 1.0 MW 690 V/Measurement of Power - Frequency2 ==
  "Power (3ph, Instantaneous)1" : powerlib_meascontrol/Measurements/Power (3ph, Instantaneous)
      settings: SourceProductName=Simscape Power Systems
  P (W) : Outport
  wires:
  [I_ac_line_2] -> "Power (3ph, Instantaneous)1"/2
  "Power (3ph, Instantaneous)1"/1 -> P (W)/1  "Pot"
  [V_ac_line_2] -> "Power (3ph, Instantaneous)1"/1

== system BESS_Voltage_Controle/BESS 1.0 MW 690 V/Measurement of Power - Frequency4 ==
  PLL (3ph)1 : powerlib_meascontrol/PLL/PLL (3ph)  Commented=on  Fmin=45  Par_Init=[0, f]  ParK=[180, 3200, 1]  TcD=1e-4  MaxRateChangeFreq=12  FilterCutOffFreq=25  Ts=0  AGC=on
  "Power (3ph, Instantaneous)1" : powerlib_meascontrol/Measurements/Power (3ph, Instantaneous)
      settings: SourceProductName=Simscape Power Systems
  F (Hz) : Outport
  P (W) : Outport  Port=2
  wires:
  [I_ac_syn_low] -> "Power (3ph, Instantaneous)1"/2
  PLL (3ph)1/1 -> F (Hz)/1
  "Power (3ph, Instantaneous)1"/1 -> P (W)/1  "Pot"
  [V_ac_syn_low] -> PLL (3ph)1/1, "Power (3ph, Instantaneous)1"/1

== system BESS_Voltage_Controle/BESS 1.0 MW 690 V/Measurement of Power - Frequency7 ==
  "Power (3ph, Instantaneous)1" : powerlib_meascontrol/Measurements/Power (3ph, Instantaneous)
      settings: SourceProductName=Simscape Power Systems
  P (W) : Outport
  wires:
  [I_ac_load] -> "Power (3ph, Instantaneous)1"/2
  "Power (3ph, Instantaneous)1"/1 -> P (W)/1  "Pot"
  [V_ac_load] -> "Power (3ph, Instantaneous)1"/1

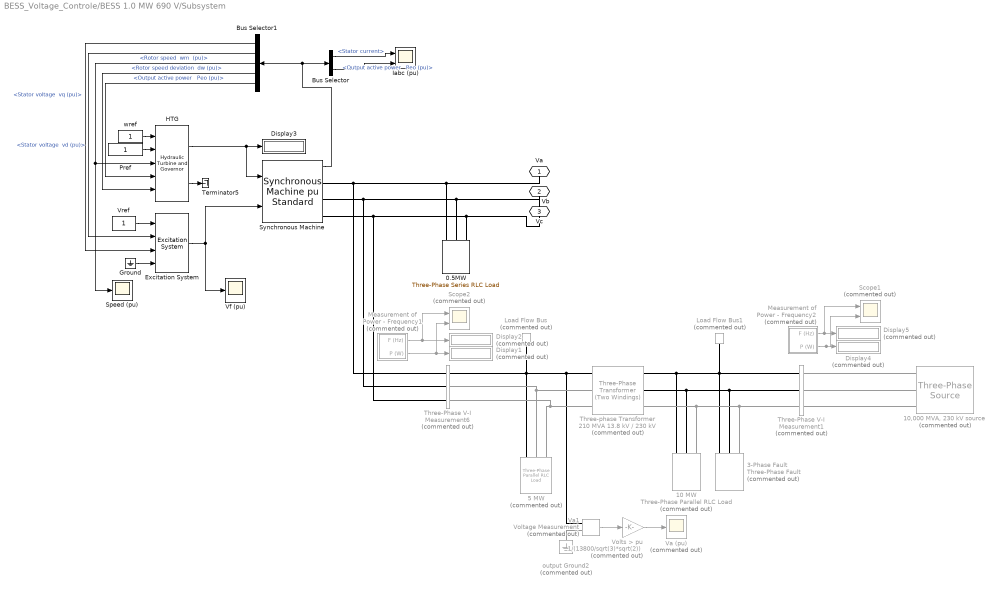
== system BESS_Voltage_Controle/BESS 1.0 MW 690 V/Subsystem ==
  " Iabc (pu)" : Scope  NumInputPorts=2
  " Speed (pu)" : Scope
  0.5MW : powerlib/Elements/Three-Phase Series RLC Load  LConnTagsString=A|B|C  Configuration=Y (grounded)  NominalVoltage=13800  Vabc=[1e3 1e3 1e3]  Vabcp=[1e3 1e3 1e3]  NominalFrequency=f  UnbalancedPower=off  ActivePower=0.5e6  InductivePower=0  CapacitivePower=0  Pabc=[10e3 9e3 11e3]  QLabc=[100 90 110]  QCabc=[100 90 110]  Pabcp=[10e3 9e3 11e3]  QLabcp=[100 90 110]  QCabcp=[100 90 110]  Measurements=None  LoadType=constant Z
  10 MW : powerlib/Elements/Three-Phase Parallel RLC Load  Commented=on  LConnTagsString=A|B|C  Configuration=Y (grounded)  NominalVoltage=230e3  Vabc=[1e3 1e3 1e3]  Vabcp=[1e3 1e3 1e3]  NominalFrequency=f  UnbalancedPower=off  ActivePower=10000000  InductivePower=0  CapacitivePower=0  Pabc=[10e3 9e3 11e3]  QLabc=[100 90 110]  QCabc=[100 90 110]  Pabcp=[10e3 9e3 11e3]  QLabcp=[100 90 110]  QCabcp=[100 90 110]  Measurements=None  LoadType=constant Z
  "10,000 MVA, 230 kV source" : powerlib/Electrical Sources/Three-Phase Source  Commented=on  InternalConnection=Yg  VoltagePhases=off  Voltage=(230000)*1.00006  PhaseAngle=-0.77547  Voltage_phases=[25e3 25e3 25e3]/sqrt(3)  PhaseAngles_phases=[0 -120 +120]  Frequency=60  NonIdealSource=on  SpecifyImpedance=on  Resistance=0.529  Inductance=0.0140  ShortCircuitLevel=10000e6  BaseVoltage=230e3  XRratio=10  BusType=swing  Pref=0  Qref=0  Prefabc=[10e3, 10e3, 10e3]  Qrefabc=[0, 0, 0]  Qmin=-Inf  Qmax=Inf
  3-Phase Fault : powerlib/Elements/Three-Phase Fault  Commented=on  InitialStates=0  FaultA=on  FaultB=on  FaultC=on  GroundFault=on  SwitchTimes=[ 0.1 0.2]  External=off  SwitchStatus=NaN  FaultResistance=1e-3  GroundResistance=1e-3  SnubberResistance=inf  SnubberCapacitance=inf  Measurements=None
  5 MW : powerlib/Elements/Three-Phase Parallel RLC Load  Commented=on  LConnTagsString=A|B|C  Configuration=Y (grounded)  NominalVoltage=13.8e3  Vabc=[1e3 1e3 1e3]  Vabcp=[1e3 1e3 1e3]  NominalFrequency=60  UnbalancedPower=off  ActivePower=5000000  InductivePower=0  CapacitivePower=0  Pabc=[10e3 9e3 11e3]  QLabc=[100 90 110]  QCabc=[100 90 110]  Pabcp=[10e3 9e3 11e3]  QLabcp=[100 90 110]  QCabcp=[100 90 110]  Measurements=None  LoadType=constant Z
  Bus Selector : BusSelector  OutputSignals="Stator current,Output active power   Peo (pu)"
  Bus Selector1 : BusSelector  OutputSignals="dq0 components.Stator voltage  vq (pu),dq0 components.Stator voltage  vd (pu),Mechanical.Rotor speed  wm  (pu),Mechanical.Rotor speed deviation  dw (pu),Output active power   Peo (pu)"
  Display{1..2,4..5} (4 alike) : Display  Commented=on
  Display3 : Display
  Excitation System : sps_avr/Excitation System  tr=20e-3  reg=[ 300, 0.001 ]  exc=[ 1, 0 ]  tgr=[ 0, 0 ]  damp=[ 0.001, 0.1 ]  sat=[ 0, 0 ]  lim=[ -11.5, 11.5, 0 ]  v0=[1,1.29071]
      settings: SourceProductName=Simscape Power Systems  SourceProductBaseCode=PS
  Ground : Ground
  HTG : powerlib/Machines/Hydraulic Turbine and Governor  sm="[ 10/3  0.07 ]"  gate="[  0.01  0.97518  -0.1  0.1 ]"  reg="[  0.05  1.163  0.105  0  0.01  ]"  hyd="[  0  2.67  ]"  dref=0  po=1
      settings: SourceProductName=Simscape Power Systems  SourceProductBaseCode=PS
  Load Flow Bus : powerlib/Measurements/Load Flow Bus  Commented=on  LConnTagsString=a  Phases=single  Connectors=on one side  ID=B1  Vbase=13.8e3  Vref=1  Vangle=0  VLF=1  VLFb=1  VLFc=1  angleLF=-23.67  angleLFb=0  angleLFc=0
      settings: AttributesFormatString=%<ID>\n%<Vbase>V\n%<VLF>pu\n%<angleLF>deg.  SourceProductName=Simscape Power Systems
  Load Flow Bus1 : powerlib/Measurements/Load Flow Bus  Commented=on  LConnTagsString=a  Phases=single  Connectors=on one side  ID=B2  Vbase=230e3  Vref=1  Vangle=0  VLF=1  VLFb=1  VLFc=1  angleLF=0  angleLFb=0  angleLFc=0
      settings: AttributesFormatString=%<ID>\n%<Vbase>V\n%<VLF>pu\n%<angleLF>deg.  SourceProductName=Simscape Power Systems
  Measurement of Power - Frequency1 : Subsystem  Commented=on
  Measurement of Power - Frequency2 : Subsystem  Commented=on
  Pref : Constant
  Scope1 : Scope  Commented=on  NumInputPorts=2
  Scope2 : Scope  Commented=on  NumInputPorts=2
  "Synchronous Machine " : powerlib/Machines/Synchronous Machine pu Standard  PresetModel=No  MechanicalLoad=Mechanical power Pm  ShowDetailedParameters=on  RotorType=Salient-pole  Units=per unit standard parameters  MeasurementBus=off  NominalParameters="[ 7.5e6  13800   f ]"  Reactances1=[ 31 32 33 34 35 36 37 ]  Reactances2=[ 1.305, 0.296, 0.252, 0.474, 0.243, 0.18 ]  dAxisTimeConstants=Short-circuit  qAxisTimeConstants=Open-circuit  TimeConstants1=[]  TimeConstants2=[]  TimeConstants3=[]  TimeConstants4=[]  TimeConstants5=[ 1.01, 0.053, 0.1 ]  TimeConstants6=[]  TimeConstants7=[]  TimeConstants8=[]  StatorResistance=2.8544e-3  Mechanical=[ 3.2 0 2]  PolePairs=2  InitialConditions=[0 -94.2826 0.750185 0.750185 0.750185 -24.943 -144.943 95.057 1.29071]  SetSaturation=off  Saturation=[0.6404,0.7127,0.8441,0.9214,0.9956,1.082,1.19,1.316,1.457;0.7,0.7698,0.8872,0.9466,0.9969,1.046,1.1,1.151,1.201]  LoadFlowParameters=[1 150000000 0 0]  TsPowergui=0  TsBlock=-1  IterativeModel=Trapezoidal non iterative  IterativeDiscreteModel=Trapezoidal non iterative  BusType=PV  Pref=150000000  Qref=0  Qmin=-Inf  Qmax=Inf  PLF=0  QLF=0
      settings: AttributesFormatString=\n\n  SourceProductName=Simscape Power Systems
  Terminator5 : Terminator
  Three-Phase V-I Measurement1 : powerlib/Measurements/Three-Phase V-I Measurement  Commented=on  VoltageMeasurement=phase-to-ground  SetLabelV=on  LabelV=V_ac_syn_low2  Vpu=off  VpuLL=off  CurrentMeasurement=yes  SetLabelI=on  LabelI=I_ac_syn_low2  Ipu=off  Pbase=100e6  Vbase=500e3  OutputType=Complex  PhasorSimulation=off  PSBequivalent=0
  Three-Phase V-I Measurement6 : powerlib/Measurements/Three-Phase V-I Measurement  Commented=on  VoltageMeasurement=phase-to-ground  SetLabelV=on  LabelV=V_ac_syn_low1  Vpu=off  VpuLL=off  CurrentMeasurement=yes  SetLabelI=on  LabelI=I_ac_syn_low1  Ipu=off  Pbase=100e6  Vbase=500e3  OutputType=Complex  PhasorSimulation=off  PSBequivalent=0
  Three-phase Transformer 210 MVA 13.8 kV / 230 kV : powerlib/Elements/Three-Phase Transformer (Two Windings)  Commented=on  Winding1Connection=Delta (D1)  Winding2Connection=Yg  CoreType=Three single-phase transformers  SetSaturation=off  Hysteresis=off  DataFile='hysteresis'  SetInitialFlux=off  Measurements=None  UNITS=pu  NominalPower=[ 210e6 60 ]  Winding1="[ 13.8e3 0.0027  0.08]"  Winding2=[ 230e3 0.0027 0.08]  Rm=500  Lm=500  L0=0.5  Saturation="[ 0,0  ;  0.005,1.2  ;  1.0,1.4 ]"  InitialFluxes=[ 0.8 , -0.8 , 0.7 ]  MoreParameters=off  BreakLoop=off  DataType=off  TransfoNumber=0
  Va (pu) : Scope  Commented=on
  Va1 : powerlib/Measurements/Voltage Measurement  Tag=PoWeRsYsTeMmEaSuReMeNt  Commented=on  PhasorSimulation=off  OutputType=Magnitude  PSBequivalent=0
  Vf (pu) : Scope
  Volts > pu : Gain  Commented=on  Gain=1/(13800/sqrt(3)*sqrt(2))  SaturateOnIntegerOverflow=on  OutDataTypeStr=Inherit: Same as input  ParamDataTypeStr=Inherit: Same as input
  Vref : Constant
  output Ground2 : powerlib/Elements/Ground  Commented=on  LConnTagsString=a
  wref : Constant
  Va : PMIOPort  Port=1  Side=Left
  Vb : PMIOPort  Port=2  Side=Left
  Vc : PMIOPort  Port=3  Side=Left
  wires:
  Bus Selector1/5 -> HTG/4  "<Output active power   Peo (pu)>"
  HTG/2 -> Terminator5/1
  Bus Selector1/3 -> HTG/3, " Speed (pu)"/1  "<Rotor speed  wm  (pu)>"
  Bus Selector/1 -> " Iabc (pu)"/1  "<Stator current>"
  Bus Selector1/2 -> Excitation System/2  "<Stator voltage  vd (pu)>"
  Ground/1 -> Excitation System/4
  Bus Selector1/1 -> Excitation System/3  "<Stator voltage  vq (pu)>"
  Va1/1 -> Volts > pu/1
  Excitation System/1 -> Vf (pu)/1, "Synchronous Machine "/2
  Bus Selector1/4 -> HTG/5  "<Rotor speed deviation  dw (pu)>"
  Volts > pu/1 -> Va (pu)/1
  Pref/1 -> HTG/2
  wref/1 -> HTG/1
  Vref/1 -> Excitation System/1
  "Synchronous Machine "/1 -> Bus Selector/1, Bus Selector1/1
  Measurement of Power - Frequency1/1(F (Hz)) -> Scope2/1, Display2/1
  Measurement of Power - Frequency1/2(P (W)) -> Scope2/2, Display1/1
  Bus Selector/2 -> " Iabc (pu)"/2  "<Output active power   Peo (pu)>"
  HTG/1 -> "Synchronous Machine "/1, Display3/1
  Measurement of Power - Frequency2/1(F (Hz)) -> Scope1/1, Display5/1
  Measurement of Power - Frequency2/2(P (W)) -> Scope1/2, Display4/1
  connections:
  Va1/LConn1 -- Three-Phase V-I Measurement6/RConn1 -- 5 MW/LConn1 -- Load Flow Bus/LConn1 -- Three-phase Transformer 210 MVA 13.8 kV / 230 kV/LConn1
  5 MW/LConn3 -- Three-Phase V-I Measurement6/RConn3 -- Three-phase Transformer 210 MVA 13.8 kV / 230 kV/LConn3
  10 MW/LConn2 -- Three-phase Transformer 210 MVA 13.8 kV / 230 kV/RConn2 -- Three-Phase V-I Measurement1/LConn2 -- 3-Phase Fault/LConn2
  Load Flow Bus1/LConn1 -- Three-phase Transformer 210 MVA 13.8 kV / 230 kV/RConn1 -- 10 MW/LConn1 -- Three-Phase V-I Measurement1/LConn1 -- 3-Phase Fault/LConn1
  3-Phase Fault/LConn3 -- Three-Phase V-I Measurement1/LConn3 -- Three-phase Transformer 210 MVA 13.8 kV / 230 kV/RConn3 -- 10 MW/LConn3
  5 MW/LConn2 -- Three-Phase V-I Measurement6/RConn2 -- Three-phase Transformer 210 MVA 13.8 kV / 230 kV/LConn2
  output Ground2/LConn1 -- Va1/LConn2
  0.5MW/LConn1 -- Three-Phase V-I Measurement6/LConn1 -- "Synchronous Machine "/RConn1 -- Va/RConn1
  Vb/RConn1 -- "Synchronous Machine "/RConn2 -- Three-Phase V-I Measurement6/LConn2 -- 0.5MW/LConn2
  0.5MW/LConn3 -- "Synchronous Machine "/RConn3 -- Three-Phase V-I Measurement6/LConn3 -- Vc/RConn1
  Three-Phase V-I Measurement1/RConn1 -- "10,000 MVA, 230 kV source"/RConn1
  Three-Phase V-I Measurement1/RConn2 -- "10,000 MVA, 230 kV source"/RConn2
  Three-Phase V-I Measurement1/RConn3 -- "10,000 MVA, 230 kV source"/RConn3

== system BESS_Voltage_Controle/BESS 1.0 MW 690 V/Subsystem1 ==
  In1 : Inport
  Bus Selector : BusSelector  OutputSignals=SOC (%),Current (A),Voltage (V)
  tag scope: I_dc_bat=global, SOC=global, V_dc_bat=global
  wires:
  Bus Selector/3 -> [V_dc_bat]  "<Voltage (V)>"
  Bus Selector/1 -> [SOC]  "<SOC (%)>"
  In1/1 -> Bus Selector/1
  Bus Selector/2 -> [I_dc_bat]  "<Current (A)>"
